simulink model "Events7"  (Simulink 6.0)
settings: Solver=ode45  StartTime=0.0  StopTime=10.0  RelTol=1e-3
settings Model: Creator=scaife  LastModifiedBy=scaife  ExtModeAutoUpdateStatusClock=off
settings DataIOCC: SignalLoggingName=sigsOut
settings DebuggingCC: SolverPrmCheckMsg=none
settings HardwareCC: TargetUnknown=on
settings STFCustomTargetCC: TargetFcnLib=ansi_tfl_tmw.mat  GenFloatMathFcnCalls=ANSI_C  ModelReferenceCompliant=off  SystemTargetFile=grt.tlc

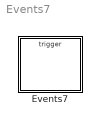
== system Events7 ==
  Events7 : Stateflow chart

== stateflow chart Events7 ==
  state T1 [parallel]
    state A
    state B
    (default) -> A
    A -> B : E
    B -> A : E
  state T2 [parallel]
    state C
    state D
    (default) -> C
    C -> D : enter(B)
    D -> C : enter(A)
  events: E input EITHER_EDGE_EVENT
